simulink model "vibration"  (R2015b)
settings: Solver=FixedStepAuto  StartTime=0.0  StopTime=60  FixedStep=1/mpu_sampling_frequency  RelTol=1e-3
values from neighbouring files (symbols this model uses):
  mpu_sampling_frequency = 819.2    [adis_imu_settings.m]    (also in imu_settings.m = 200)
libraries: simulink x1
settings Model: Creator=TOOsab  LastModifiedBy=TOOsab

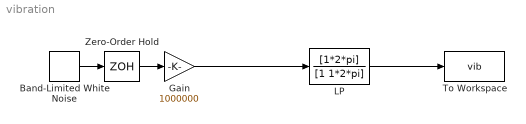
== system vibration ==
  Band-Limited White Noise : simulink/Sources/Band-Limited White Noise  Cov=[1000]  Ts=1/mpu_sampling_frequency  seed=[23341]
  Gain : Gain  Gain=1000000
  LP : TransferFcn  Numerator=[1*2*pi]  Denominator=[1 1*2*pi]
  To Workspace : ToWorkspace  VariableName=vib  SampleTime=-1
  Zero-Order Hold : ZeroOrderHold  SampleTime=1/mpu_sampling_frequency
  wires:
  Band-Limited White Noise/1 -> Zero-Order Hold/1
  Zero-Order Hold/1 -> Gain/1
  Gain/1 -> LP/1
  LP/1 -> To Workspace/1
